simulink library "friction_coeff2clq"  (R2018b)
settings: Solver=ode45  StartTime=0.0  StopTime=10.0  RelTol=1e-3  EnableMultiTasking=on
libraries: carnot x1
settings Model: Creator=lena.frank  LastModifiedBy=P41573
settings DataIOCC: LimitDataPoints=on  SaveFormat=Array  SignalLoggingSaveFormat=ModelDataLogs
settings OptimizationCC: ExpressionDepthLimit=2147483647  LifeSpan=inf
settings DebuggingCC: UnderspecifiedInitializationDetection=Classic  MergeDetectMultiDrivingBlocksExec=none  SolverPrmCheckMsg=warning  FcnCallInpInsideContextMsg=warning  StateNameClashWarn=warning  SFUnexpectedBacktrackingDiag=warning  SFNoUnconditionalDefaultTransitionDiag=warning  SFExecutionAtInitializationDiag=none
settings HardwareCC: ProdBitPerPointer=32  ProdBitPerSizeT=32  ProdBitPerPtrDiffT=32  ProdLargestAtomicFloat=None  ProdIntDivRoundTo=Undefined  ProdEndianess=Unspecified  ProdWordSize=32  ProdHWDeviceType=32-bit Generic
settings ModelReferenceCC: PropagateSignalLabelsOutOfModel=off
settings SFSimCC: SimUseLocalCustomCode=off
settings RTWCC: RTWUseLocalCustomCode=off
settings CodeAppCC: StateflowObjectComments=on
settings GRTTargetCC: TargetLangStandard=C89/C90 (ANSI)  GeneratePreprocessorConditionals=Disable all  CombineOutputUpdateFcns=off  GRTInterface=on
settings ConfigComp: CovMetricSettings=dw  CovHtmlReporting=on  CovSaveCumulativeToWorkspaceVar=on  CovSaveSingleToWorkspaceVar=on  CovExternalEMLEnable=off

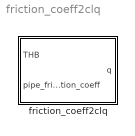
== system friction_coeff2clq ==
  friction_coeff2clq : Subsystem  mask(friction coefficient 2 clq){Value=0.05, Gain=1}
      mask prompts: Value "Diameter of pipe in m"; Gain "Pipe length in m"
      mask help:
      | Determine the clq coefficients from pipe friction coefficent lambda:
      | dp = lambda * length * denstiy / (dia * 2) * v^2
      | for round pipes:
      | dp  = 8 * lambda * l * mdot^2 / (rho * pi^2 * dia^5)
      | Carnot pressure drop calculation:
      | dp = c + l*mdot + q*mdot^2
      | so:  q = 8 * lambda * l / (rho * pi^2 * dia^5)
      | and l = 0; c = 0;
      mask TypeOptions Value: diameter/Value
      mask TypeOptions Gain: length/Gain

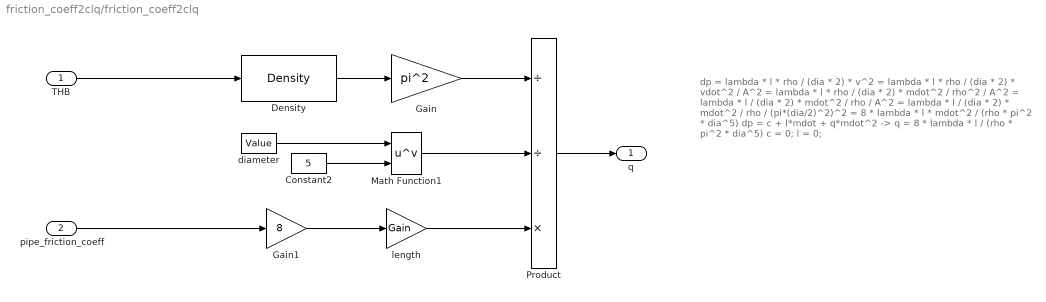
== system friction_coeff2clq/friction_coeff2clq ==
  note: dp = lambda * l * rho / (dia * 2) * v^2
      |    = lambda * l * rho / (dia * 2) * vdot^2 / A^2
      |     = lambda * l * rho / (dia * 2) * mdot^2 / rho^2 / A^2
      |     = lambda * l / (dia * 2) * mdot^2 / rho / A^2
      |     = lambda * l / (dia * 2) * mdot^2 / rho / (pi*(dia/2)^2)^2
      |     = 8 * lambda * l * mdot^2 / (rho * pi^2 * dia^5)
      |
      | dp = c + l*mdot + q*mdot^2
      |
      | -> q = 8 * lambda * l / (rho * pi^2 * dia^5)
      | c = 0; l = 0;
  THB : Inport
  pipe_friction_coeff : Inport  Port=2
  Constant2 : Constant  Value=5
  Density : carnot/Basic/Material_Properties/Density  VariantControl=CarlibClassic  INPUTARGUMENTS=THB  DEBUGLEVEL=DEBUGLEVEL  MAXTOTALWARNINGS=inf  MAXCONSECUTIVEWARNINGS=inf  WRITETOFILE=0  FILENAME='errors.txt'
      settings: SourceProductName=Carnot
  Gain : Gain  Gain=pi^2
  Gain1 : Gain  Gain=8
  Math Function1 : Math  Operator=pow  SaturateOnIntegerOverflow=on
  Product : Product  Inputs=//*  RndMeth=Zero
  diameter : Constant  Value=Value
  length : Gain  Gain=Gain
  q : Outport
  wires:
  length/1 -> Product/3
  Constant2/1 -> Math Function1/2
  diameter/1 -> Math Function1/1
  Gain1/1 -> length/1
  pipe_friction_coeff/1 -> Gain1/1
  Math Function1/1 -> Product/2
  Density/1 -> Gain/1
  THB/1 -> Density/1
  Gain/1 -> Product/1
  Product/1 -> q/1
